simulink model "base_model_1_new_Copy_restored_from_autosave"  (R2025b)
settings: Solver=FixedStepAuto  StartTime=60  StopTime=36000  RelTol=1e-3
settings Model: Creator=Gmusl  LastModifiedBy=caddo

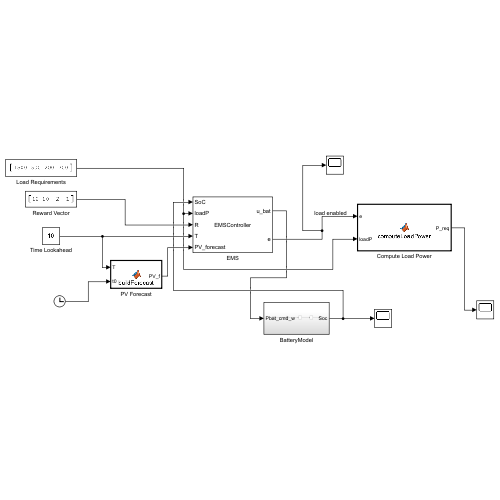
[thumbnail: Simulink's stored preview of the top-level diagram]
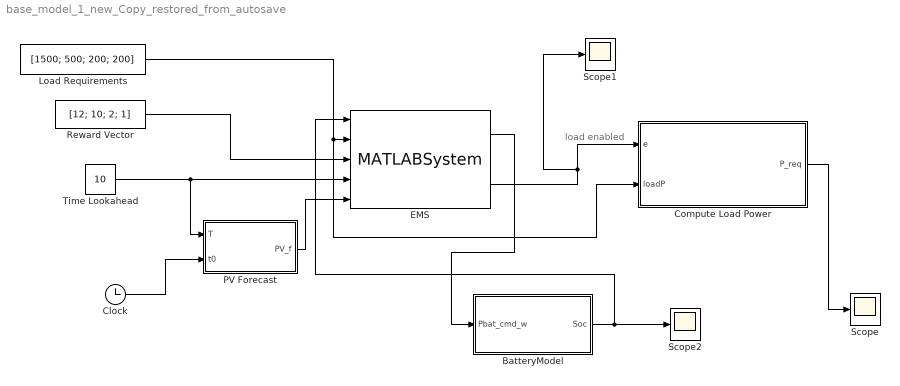
== system base_model_1_new_Copy_restored_from_autosave ==
  note: load enabled
  BatteryModel : Subsystem
  Clock : Clock
  Compute Load Power : MATLAB Function  TreatAsAtomicUnit=on
  EMS : MATLABSystem  System=EMSController  SimulateUsing=Code generation
      mask Type: EMSController
  Load Requirements : Constant  Value=[1500; 500; 200; 200]
  PV Forecast : MATLAB Function  TreatAsAtomicUnit=on
  Reward Vector : Constant  Value=[12; 10; 2; 1]
  Scope : Scope
  Scope1 : Scope
  Scope2 : Scope
      settings: DataLoggingVariableName=ScopeData2
  Time Lookahead : Constant  Value=10
  wires:
  BatteryModel/1(Soc) -> EMS/1, Scope2/1
  Time Lookahead/1 -> EMS/4, PV Forecast/1(T)
  Load Requirements/1 -> Compute Load Power/2(loadP), EMS/2
  Reward Vector/1 -> EMS/3
  PV Forecast/1(PV_f) -> EMS/5
  EMS/1 -> BatteryModel/1(Pbat_cmd_w)
  EMS/2 -> Scope1/1, Compute Load Power/1(e)
  Compute Load Power/1(P_req) -> Scope/1
  Clock/1 -> PV Forecast/2(t0)

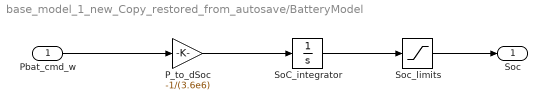
== system base_model_1_new_Copy_restored_from_autosave/BatteryModel ==
  Pbat_cmd_w : Inport
  P_to_dSoc : Gain  Gain=-1/(3.6e6)
  SoC_integrator : Integrator  InitialCondition=0.8
  Soc_limits : Saturate  UpperLimit=0.95  LowerLimit=0.2
  Soc : Outport
  wires:
  Pbat_cmd_w/1 -> P_to_dSoc/1
  P_to_dSoc/1 -> SoC_integrator/1
  SoC_integrator/1 -> Soc_limits/1
  Soc_limits/1 -> Soc/1

== matlab function base_model_1_new_Copy_restored_from_autosave/PV Forecast ==
  data: T input; PV_f output; t0 input
function PV_f = buildForecast(T, t0)
%#codegen

% timestep (seconds) – match your fixed-step size
dt = 60; 

% PV model parameters
Pmax = 2000; 
day_length = 86400; 

PV_f = zeros(T,1);

for k = 1:T
    t_future = t0 + k*dt;
    PV_f(k) = max(Pmax * sin(pi * t_future / day_length), 0);
end

== matlab function base_model_1_new_Copy_restored_from_autosave/Compute Load Power ==
  data: e input; P_req output; loadP input
function P_req = computeLoadPower(e, loadP)
% e      : vector of enable signals (0/1)
% loadP  : vector of load power ratings (W)
% Output : total required load power (W)

    % Ensure column vectors
    e = e(:);
    loadP = loadP(:);

    % Total load power
    P_req = sum(e .* loadP);
end
